simulink library "variable_load_lib"  (R2012b)
settings: Solver=ode45  StartTime=0.0  StopTime=10.0  RelTol=1e-3
libraries: powerlib x6
settings Model: Creator=CH24070  LastModifiedBy=CH24070

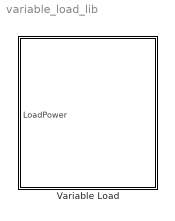
== system variable_load_lib ==
  Variable Load : Subsystem

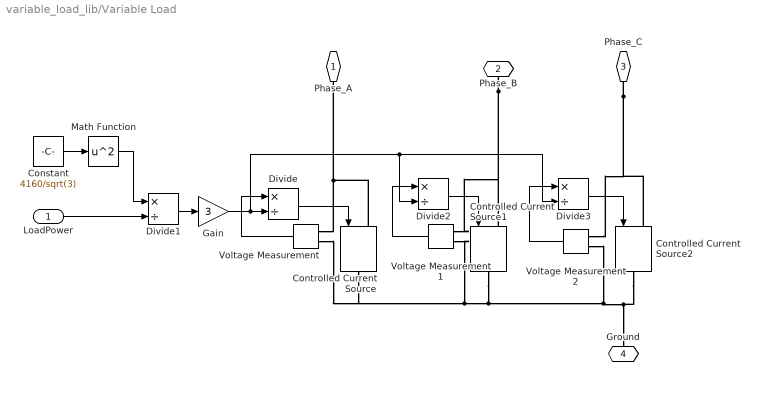
== system variable_load_lib/Variable Load ==
  LoadPower : Inport
  Constant : Constant  Value=4160/sqrt(3)
  Controlled Current Source : powerlib/Electrical Sources/Controlled Current Source  Initialize=on  Source_Type=AC  Amplitude=0  Phase=0  Frequency=0  Measurements=None
  Controlled Current Source1 : powerlib/Electrical Sources/Controlled Current Source  Initialize=on  Source_Type=AC  Amplitude=0  Phase=0  Frequency=0  Measurements=None
  Controlled Current Source2 : powerlib/Electrical Sources/Controlled Current Source  Initialize=on  Source_Type=AC  Amplitude=0  Phase=0  Frequency=0  Measurements=None
  Divide{,1..3} (4 alike) : Product  Inputs=*/
  Gain : Gain  Gain=3
  Math Function : Math  Operator=square  SaturateOnIntegerOverflow=on
  Voltage Measurement : powerlib/Measurements/Voltage Measurement  PhasorSimulation=off  OutputType=Complex  PSBequivalent=0
  Voltage Measurement1 : powerlib/Measurements/Voltage Measurement  PhasorSimulation=off  OutputType=Complex  PSBequivalent=0
  Voltage Measurement2 : powerlib/Measurements/Voltage Measurement  PhasorSimulation=off  OutputType=Complex  PSBequivalent=0
  Phase_A : PMIOPort  Port=1  Side=Right
  Phase_B : PMIOPort  Port=2  Side=Right
  Phase_C : PMIOPort  Port=3  Side=Right
  Ground : PMIOPort  Port=4  Side=Right
  wires:
  Math Function/1 -> Divide1/1
  Gain/1 -> Divide/2, Divide2/2, Divide3/2
  Voltage Measurement/1 -> Divide/1
  Divide/1 -> Controlled Current Source/1
  Voltage Measurement2/1 -> Divide3/1
  Divide3/1 -> Controlled Current Source2/1
  Divide1/1 -> Gain/1
  Constant/1 -> Math Function/1
  Voltage Measurement1/1 -> Divide2/1
  Divide2/1 -> Controlled Current Source1/1
  LoadPower/1 -> Divide1/2
  connections:
  Phase_C/RConn1 -- Voltage Measurement2/LConn1 -- Controlled Current Source2/LConn1
  Phase_B/RConn1 -- Voltage Measurement1/LConn1 -- Controlled Current Source1/LConn1
  Controlled Current Source2/RConn1 -- Voltage Measurement2/LConn2 -- Controlled Current Source1/RConn1 -- Controlled Current Source/RConn1 -- Voltage Measurement/LConn2 -- Voltage Measurement1/LConn2 -- Ground/RConn1
  Controlled Current Source/LConn1 -- Phase_A/RConn1 -- Voltage Measurement/LConn1
